simulink model "Full_load_sim_doc"  (R2020a)
settings: Solver=VariableStepAuto  StartTime=0.0  StopTime=50000  RelTol=1e-3
values from neighbouring files (symbols this model uses):
  BlySyreON = 1    [sim_starter.m]
  LiIonLilleON = 1    [sim_starter.m]
  LiIonStorON = 1    [sim_starter.m]
  LoadBlySyre = load    [sim_starter.m]
  LoadLille = load    [sim_starter.m]
  LoadLiStor = 0    [sim_starter.m]
  LoadNiMH = load    [sim_starter.m]
  LoadSaltVand = load    [sim_starter.m]
  NiMHON = 1    [sim_starter.m]
  SaltVandON = 1    [sim_starter.m]
undefined symbols (not defined in the file or in its folder): Hydride, Metal, Nickel
libraries: nesl_utility x28, fl_lib x24, powerlib x4, ee_lib x4, electricdrivelib x1
(part 1 of 2)
settings Model: PacingRate=0.100000  Creator=Philip AMH  LastModifiedBy=jenslawl
settings SolverCC: ZeroCrossAlgorithm=Adaptive  AlgebraicLoopSolver=LineSearch
settings OptimizationCC: DefaultParameterBehavior=Inlined  UseDivisionForNetSlopeComputation=on  GainParamInheritBuiltInType=on  UseFloatMulNetSlope=on  InlineInvariantSignals=on  EnhancedBackFolding=on  BooleansAsBitfields=on  PassReuseOutputArgsAs=Individual arguments  StateBitsets=on  DataBitsets=on  ZeroExternalMemoryAtStartup=off  ZeroInternalMemoryAtStartup=off  NoFixptDivByZeroProtection=on  EfficientFloat2IntCast=on  LifeSpan=1  OptimizeBlockOrder=speed  DifferentSizesBufferReuse=on  EfficientTunableParamExpr=on
settings DebuggingCC: IgnoredZcDiagnostic=none  ParameterTunabilityLossMsg=error
settings SFSimCC: MATLABDynamicMemAlloc=off
settings RTWCC: SystemTargetFile=ert.tlc  TemplateMakefile=ert_default_tmf  TargetLang=C++
settings CodeAppCC: ForceParamTrailComments=on  IgnoreCustomStorageClasses=off  OperatorAnnotations=on  SimulinkDataObjDesc=on  SFDataObjDesc=on  CustomSymbolStrGlobalVar=rt$N$M  CustomSymbolStrType=$N$M  CustomSymbolStrFcn=$N$M$F  CustomSymbolStrMacro=$N$M  InsertBlockDesc=on
settings ERTTargetCC: TargetLangStandard=C++03 (ISO)  GenerateSampleERTMain=on  IncludeMdlTerminateFcn=off  CombineSignalStateStructs=on  SupportAbsoluteTime=off  SupportComplex=off  SupportContinuousTime=on  InlinedParameterPlacement=NonHierarchical  RootIOFormat=Structure reference  ERTCustomFileTemplate=example_file_process.tlc  ERTFilePackagingFormat=CompactWithDataFile

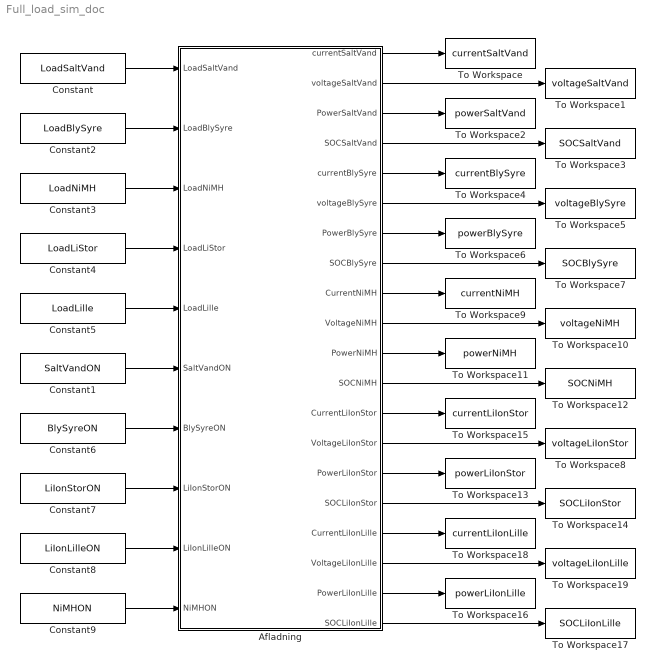
== system Full_load_sim_doc ==
  Afladning : Subsystem
  Constant : Constant  Value=LoadSaltVand
  Constant1 : Constant  Value=SaltVandON
  Constant2 : Constant  Value=LoadBlySyre
  Constant3 : Constant  Value=LoadNiMH
  Constant4 : Constant  Value=LoadLiStor
  Constant5 : Constant  Value=LoadLille
  Constant6 : Constant  Value=BlySyreON
  Constant7 : Constant  Value=LiIonStorON
  Constant8 : Constant  Value=LiIonLilleON
  Constant9 : Constant  Value=NiMHON
  To Workspace : ToWorkspace  VariableName=currentSaltVand  SampleTime=-1
  To Workspace1 : ToWorkspace  VariableName=voltageSaltVand  SampleTime=-1
  To Workspace10 : ToWorkspace  VariableName=voltageNiMH  SampleTime=-1
  To Workspace11 : ToWorkspace  VariableName=powerNiMH  SampleTime=-1
  To Workspace12 : ToWorkspace  VariableName=SOCNiMH  SampleTime=-1
  To Workspace13 : ToWorkspace  VariableName=powerLiIonStor  SampleTime=-1
  To Workspace14 : ToWorkspace  VariableName=SOCLiIonStor  SampleTime=-1
  To Workspace15 : ToWorkspace  VariableName=currentLiIonStor  SampleTime=-1
  To Workspace16 : ToWorkspace  VariableName=powerLiIonLille  SampleTime=-1
  To Workspace17 : ToWorkspace  VariableName=SOCLiIonLille  SampleTime=-1
  To Workspace18 : ToWorkspace  VariableName=currentLiIonLille  SampleTime=-1
  To Workspace19 : ToWorkspace  VariableName=voltageLiIonLille  SampleTime=-1
  To Workspace2 : ToWorkspace  VariableName=powerSaltVand  SampleTime=-1
  To Workspace3 : ToWorkspace  VariableName=SOCSaltVand  SampleTime=-1
  To Workspace4 : ToWorkspace  VariableName=currentBlySyre  SampleTime=-1
  To Workspace5 : ToWorkspace  VariableName=voltageBlySyre  SampleTime=-1
  To Workspace6 : ToWorkspace  VariableName=powerBlySyre  SampleTime=-1
  To Workspace7 : ToWorkspace  VariableName=SOCBlySyre  SampleTime=-1
  To Workspace8 : ToWorkspace  VariableName=voltageLiIonStor  SampleTime=-1
  To Workspace9 : ToWorkspace  VariableName=currentNiMH  SampleTime=-1
  wires:
  Constant/1 -> Afladning/1(LoadSaltVand)
  Constant2/1 -> Afladning/2(LoadBlySyre)
  Constant3/1 -> Afladning/3(LoadNiMH)
  Constant4/1 -> Afladning/4(LoadLiStor)
  Constant5/1 -> Afladning/5(LoadLille)
  Constant1/1 -> Afladning/6(SaltVandON)
  Constant6/1 -> Afladning/7(BlySyreON)
  Constant7/1 -> Afladning/8(LiIonStorON)
  Constant8/1 -> Afladning/9(LiIonLilleON)
  Constant9/1 -> Afladning/10(NiMHON)
  Afladning/1(currentSaltVand) -> To Workspace/1
  Afladning/3(PowerSaltVand) -> To Workspace2/1
  Afladning/2(voltageSaltVand) -> To Workspace1/1
  Afladning/4(SOCSaltVand) -> To Workspace3/1
  Afladning/8(SOCBlySyre) -> To Workspace7/1
  Afladning/6(voltageBlySyre) -> To Workspace5/1
  Afladning/5(currentBlySyre) -> To Workspace4/1
  Afladning/7(PowerBlySyre) -> To Workspace6/1
  Afladning/9(CurrentNiMH) -> To Workspace9/1
  Afladning/12(SOCNiMH) -> To Workspace12/1
  Afladning/11(PowerNiMH) -> To Workspace11/1
  Afladning/10(VoltageNiMH) -> To Workspace10/1
  Afladning/16(SOCLiIonStor) -> To Workspace14/1
  Afladning/14(VoltageLiIonStor) -> To Workspace8/1
  Afladning/13(CurrentLiIonStor) -> To Workspace15/1
  Afladning/15(PowerLiIonStor) -> To Workspace13/1
  Afladning/18(VoltageLiIonLille) -> To Workspace19/1
  Afladning/20(SOCLiIonLille) -> To Workspace17/1
  Afladning/17(CurrentLiIonLille) -> To Workspace18/1
  Afladning/19(PowerLiIonLille) -> To Workspace16/1

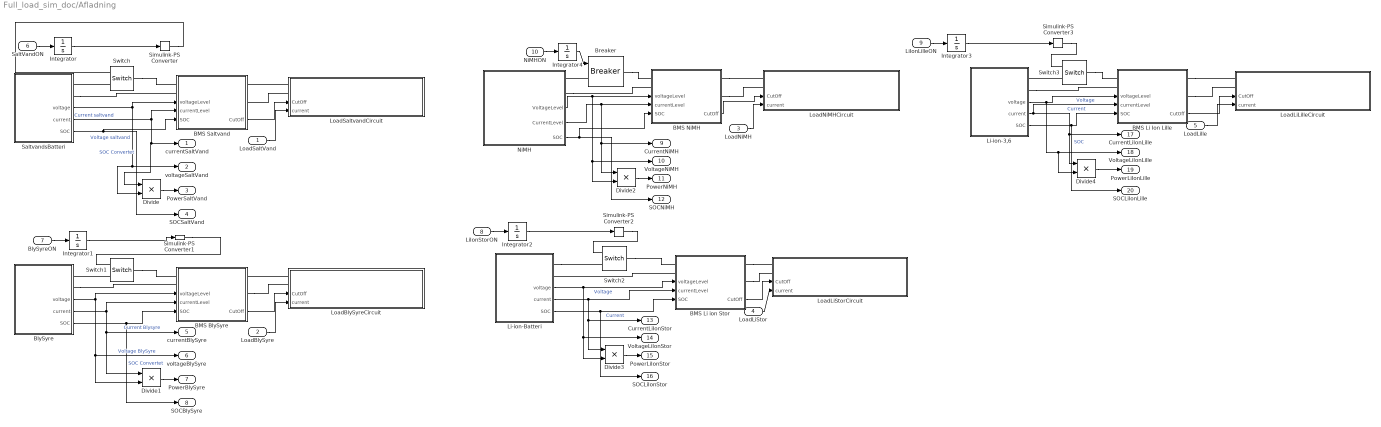
== system Full_load_sim_doc/Afladning ==
  LoadSaltVand : Inport
  LoadBlySyre : Inport  Port=2
  LoadNiMH : Inport  Port=3
  LoadLiStor : Inport  Port=4
  LoadLille : Inport  Port=5
  SaltVandON : Inport  Port=6
  BlySyreON : Inport  Port=7
  LiIonStorON : Inport  Port=8
  LiIonLilleON : Inport  Port=9
  NiMHON : Inport  Port=10
  BMS BlySyre : Subsystem
      settings: PortSchema="{\"entries\":[{\"content\":{\"sides\":[{\"content\":{\"connectorIds\":[\"LConn1\",\"LConn2\",\"In1\",\"In2\",\"In3\"]},\"type\":\"ConnectorPlacement.EquallySpacedRectSide\",\"uuid\":\"8e5b19d5-26fd-4308-a068-31d3a7110353\"},{\"content\":{\"connectorIds\":[\"RConn1\",\"RConn2\",\"Out1\"],\"side\":\"RIGHT\"},\"type\":\"ConnectorPlacement.EquallySpacedRectSide\",\"uuid\":\"43c00b24-a96d-45dd-baf7-73862471a89e\"},{\"content\":{\"connectorIds\":[],\"side\":\"TOP\"},\"type\":\"ConnectorPlacement.EquallySpacedRectSide\",\"uuid\":\"aec9a084-a9ff-4300-b99c-89bc23ebac6c\"}]},\"type\":\"ConnectorPlacement.EquallySpacedConnector\",\"uuid\":\"d767dd7e-ef5e-469c-820c-a4f5797d1fb9\"}],\"packageUris\":[\"http://schema.mathworks.com/mf0/Connector/19700101\"],\"version\":\"1.0\"}"
  BMS Li Ion Lille : Subsystem
      settings: PortSchema="{\"entries\":[{\"content\":{\"sides\":[{\"content\":{\"connectorIds\":[\"LConn1\",\"LConn2\",\"In1\",\"In2\",\"In3\"]},\"type\":\"ConnectorPlacement.EquallySpacedRectSide\",\"uuid\":\"8e5b19d5-26fd-4308-a068-31d3a7110353\"},{\"content\":{\"connectorIds\":[\"RConn1\",\"RConn2\",\"Out1\"],\"side\":\"RIGHT\"},\"type\":\"ConnectorPlacement.EquallySpacedRectSide\",\"uuid\":\"43c00b24-a96d-45dd-baf7-73862471a89e\"},{\"content\":{\"connectorIds\":[],\"side\":\"TOP\"},\"type\":\"ConnectorPlacement.EquallySpacedRectSide\",\"uuid\":\"aec9a084-a9ff-4300-b99c-89bc23ebac6c\"}]},\"type\":\"ConnectorPlacement.EquallySpacedConnector\",\"uuid\":\"d767dd7e-ef5e-469c-820c-a4f5797d1fb9\"}],\"packageUris\":[\"http://schema.mathworks.com/mf0/Connector/19700101\"],\"version\":\"1.0\"}"
  BMS Li ion Stor : Subsystem
      settings: PortSchema="{\"entries\":[{\"content\":{\"sides\":[{\"content\":{\"connectorIds\":[\"LConn1\",\"LConn2\",\"In1\",\"In2\",\"In3\"]},\"type\":\"ConnectorPlacement.EquallySpacedRectSide\",\"uuid\":\"8e5b19d5-26fd-4308-a068-31d3a7110353\"},{\"content\":{\"connectorIds\":[\"RConn1\",\"RConn2\",\"Out1\"],\"side\":\"RIGHT\"},\"type\":\"ConnectorPlacement.EquallySpacedRectSide\",\"uuid\":\"43c00b24-a96d-45dd-baf7-73862471a89e\"},{\"content\":{\"connectorIds\":[],\"side\":\"TOP\"},\"type\":\"ConnectorPlacement.EquallySpacedRectSide\",\"uuid\":\"aec9a084-a9ff-4300-b99c-89bc23ebac6c\"}]},\"type\":\"ConnectorPlacement.EquallySpacedConnector\",\"uuid\":\"d767dd7e-ef5e-469c-820c-a4f5797d1fb9\"}],\"packageUris\":[\"http://schema.mathworks.com/mf0/Connector/19700101\"],\"version\":\"1.0\"}"
  BMS NiMH : Subsystem
      settings: PortSchema="{\"entries\":[{\"content\":{\"sides\":[{\"content\":{\"connectorIds\":[\"LConn1\",\"LConn2\",\"In1\",\"In2\",\"In3\"]},\"type\":\"ConnectorPlacement.EquallySpacedRectSide\",\"uuid\":\"8e5b19d5-26fd-4308-a068-31d3a7110353\"},{\"content\":{\"connectorIds\":[\"RConn1\",\"RConn2\",\"Out1\"],\"side\":\"RIGHT\"},\"type\":\"ConnectorPlacement.EquallySpacedRectSide\",\"uuid\":\"43c00b24-a96d-45dd-baf7-73862471a89e\"},{\"content\":{\"connectorIds\":[],\"side\":\"TOP\"},\"type\":\"ConnectorPlacement.EquallySpacedRectSide\",\"uuid\":\"aec9a084-a9ff-4300-b99c-89bc23ebac6c\"}]},\"type\":\"ConnectorPlacement.EquallySpacedConnector\",\"uuid\":\"d767dd7e-ef5e-469c-820c-a4f5797d1fb9\"}],\"packageUris\":[\"http://schema.mathworks.com/mf0/Connector/19700101\"],\"version\":\"1.0\"}"
  "BMS Saltvand " : Subsystem
      settings: PortSchema="{\"entries\":[{\"content\":{\"sides\":[{\"content\":{\"connectorIds\":[\"LConn1\",\"LConn2\",\"In1\",\"In2\",\"In3\"]},\"type\":\"ConnectorPlacement.EquallySpacedRectSide\",\"uuid\":\"8e5b19d5-26fd-4308-a068-31d3a7110353\"},{\"content\":{\"connectorIds\":[\"RConn1\",\"RConn2\",\"Out1\"],\"side\":\"RIGHT\"},\"type\":\"ConnectorPlacement.EquallySpacedRectSide\",\"uuid\":\"43c00b24-a96d-45dd-baf7-73862471a89e\"},{\"content\":{\"connectorIds\":[],\"side\":\"TOP\"},\"type\":\"ConnectorPlacement.EquallySpacedRectSide\",\"uuid\":\"aec9a084-a9ff-4300-b99c-89bc23ebac6c\"}]},\"type\":\"ConnectorPlacement.EquallySpacedConnector\",\"uuid\":\"d767dd7e-ef5e-469c-820c-a4f5797d1fb9\"}],\"packageUris\":[\"http://schema.mathworks.com/mf0/Connector/19700101\"],\"version\":\"1.0\"}"
  BlySyre : Subsystem
      settings: PortSchema="{\"entries\":[{\"content\":{\"sides\":[{\"content\":{\"connectorIds\":[]},\"type\":\"ConnectorPlacement.EquallySpacedRectSide\",\"uuid\":\"b7adcffb-368c-467a-b339-3146d53f89f7\"},{\"content\":{\"connectorIds\":[\"RConn1\",\"RConn2\",\"Out1\",\"Out2\",\"Out3\"],\"side\":\"RIGHT\"},\"type\":\"ConnectorPlacement.EquallySpacedRectSide\",\"uuid\":\"78fa0dc6-8b86-442a-9e1f-c20c2cc39690\"},{\"content\":{\"connectorIds\":[],\"side\":\"TOP\"},\"type\":\"ConnectorPlacement.EquallySpacedRectSide\",\"uuid\":\"02b6bb54-52f8-4387-9821-90c0e82d6c22\"}]},\"type\":\"ConnectorPlacement.EquallySpacedConnector\",\"uuid\":\"f2eebdbf-49bd-409e-a7c0-76b4bde01873\"}],\"packageUris\":[\"http://schema.mathworks.com/mf0/Connector/19700101\"],\"version\":\"1.0\"}"
  Breaker : powerlib/Elements/Breaker  InitialState=0  SwitchingTimes="[1/60  5/60]"  External=on  BreakerResistance=0.01  SnubberResistance=1e6  SnubberCapacitance=inf  Measurements=None  MoreParameters=on  NoBreakLoop=off
  Divide{,1..4} (5 alike) : Product  Inputs=**
  Integrator{,1..4} (5 alike) : Integrator
  Li-ion-3,6 : Subsystem
      settings: PortSchema="{\"entries\":[{\"content\":{\"sides\":[{\"content\":{\"connectorIds\":[]},\"type\":\"ConnectorPlacement.EquallySpacedRectSide\",\"uuid\":\"b7adcffb-368c-467a-b339-3146d53f89f7\"},{\"content\":{\"connectorIds\":[\"RConn1\",\"RConn2\",\"Out1\",\"Out2\",\"Out3\"],\"side\":\"RIGHT\"},\"type\":\"ConnectorPlacement.EquallySpacedRectSide\",\"uuid\":\"78fa0dc6-8b86-442a-9e1f-c20c2cc39690\"},{\"content\":{\"connectorIds\":[],\"side\":\"TOP\"},\"type\":\"ConnectorPlacement.EquallySpacedRectSide\",\"uuid\":\"02b6bb54-52f8-4387-9821-90c0e82d6c22\"}]},\"type\":\"ConnectorPlacement.EquallySpacedConnector\",\"uuid\":\"f2eebdbf-49bd-409e-a7c0-76b4bde01873\"}],\"packageUris\":[\"http://schema.mathworks.com/mf0/Connector/19700101\"],\"version\":\"1.0\"}"
  Li-ion-Batteri : Subsystem
      settings: PortSchema="{\"entries\":[{\"content\":{\"sides\":[{\"content\":{\"connectorIds\":[]},\"type\":\"ConnectorPlacement.EquallySpacedRectSide\",\"uuid\":\"b7adcffb-368c-467a-b339-3146d53f89f7\"},{\"content\":{\"connectorIds\":[\"RConn1\",\"RConn2\",\"Out1\",\"Out2\",\"Out3\"],\"side\":\"RIGHT\"},\"type\":\"ConnectorPlacement.EquallySpacedRectSide\",\"uuid\":\"78fa0dc6-8b86-442a-9e1f-c20c2cc39690\"},{\"content\":{\"connectorIds\":[],\"side\":\"TOP\"},\"type\":\"ConnectorPlacement.EquallySpacedRectSide\",\"uuid\":\"02b6bb54-52f8-4387-9821-90c0e82d6c22\"}]},\"type\":\"ConnectorPlacement.EquallySpacedConnector\",\"uuid\":\"f2eebdbf-49bd-409e-a7c0-76b4bde01873\"}],\"packageUris\":[\"http://schema.mathworks.com/mf0/Connector/19700101\"],\"version\":\"1.0\"}"
  LoadBlySyreCircuit : Subsystem
      settings: PortSchema="{\"entries\":[{\"content\":{\"sides\":[{\"content\":{\"connectorIds\":[\"LConn1\",\"LConn2\",\"In1\",\"In2\"]},\"type\":\"ConnectorPlacement.EquallySpacedRectSide\",\"uuid\":\"b5cadee7-2d01-46ee-bf49-69402e8f136b\"},{\"content\":{\"connectorIds\":[],\"side\":\"RIGHT\"},\"type\":\"ConnectorPlacement.EquallySpacedRectSide\",\"uuid\":\"c93f53f5-1213-453b-bd10-619be19bd60a\"},{\"content\":{\"connectorIds\":[],\"side\":\"TOP\"},\"type\":\"ConnectorPlacement.EquallySpacedRectSide\",\"uuid\":\"b4015440-ddf2-46e7-8a1d-8162baf69575\"}]},\"type\":\"ConnectorPlacement.EquallySpacedConnector\",\"uuid\":\"d9e17d4e-0efd-4077-956a-1911f70d4ae6\"}],\"packageUris\":[\"http://schema.mathworks.com/mf0/Connector/19700101\"],\"version\":\"1.0\"}"
  LoadLiLilleCircuit : Subsystem
      settings: PortSchema="{\"entries\":[{\"content\":{\"sides\":[{\"content\":{\"connectorIds\":[\"LConn1\",\"LConn2\",\"In1\",\"In2\"]},\"type\":\"ConnectorPlacement.EquallySpacedRectSide\",\"uuid\":\"b5cadee7-2d01-46ee-bf49-69402e8f136b\"},{\"content\":{\"connectorIds\":[],\"side\":\"RIGHT\"},\"type\":\"ConnectorPlacement.EquallySpacedRectSide\",\"uuid\":\"c93f53f5-1213-453b-bd10-619be19bd60a\"},{\"content\":{\"connectorIds\":[],\"side\":\"TOP\"},\"type\":\"ConnectorPlacement.EquallySpacedRectSide\",\"uuid\":\"b4015440-ddf2-46e7-8a1d-8162baf69575\"}]},\"type\":\"ConnectorPlacement.EquallySpacedConnector\",\"uuid\":\"d9e17d4e-0efd-4077-956a-1911f70d4ae6\"}],\"packageUris\":[\"http://schema.mathworks.com/mf0/Connector/19700101\"],\"version\":\"1.0\"}"
  LoadLiStorCircuit : Subsystem
      settings: PortSchema="{\"entries\":[{\"content\":{\"sides\":[{\"content\":{\"connectorIds\":[\"LConn1\",\"LConn2\",\"In1\",\"In2\"]},\"type\":\"ConnectorPlacement.EquallySpacedRectSide\",\"uuid\":\"b5cadee7-2d01-46ee-bf49-69402e8f136b\"},{\"content\":{\"connectorIds\":[],\"side\":\"RIGHT\"},\"type\":\"ConnectorPlacement.EquallySpacedRectSide\",\"uuid\":\"c93f53f5-1213-453b-bd10-619be19bd60a\"},{\"content\":{\"connectorIds\":[],\"side\":\"TOP\"},\"type\":\"ConnectorPlacement.EquallySpacedRectSide\",\"uuid\":\"b4015440-ddf2-46e7-8a1d-8162baf69575\"}]},\"type\":\"ConnectorPlacement.EquallySpacedConnector\",\"uuid\":\"d9e17d4e-0efd-4077-956a-1911f70d4ae6\"}],\"packageUris\":[\"http://schema.mathworks.com/mf0/Connector/19700101\"],\"version\":\"1.0\"}"
  LoadNiMHCircuit : Subsystem
      settings: PortSchema="{\"entries\":[{\"content\":{\"sides\":[{\"content\":{\"connectorIds\":[\"LConn1\",\"LConn2\",\"In1\",\"In2\"]},\"type\":\"ConnectorPlacement.EquallySpacedRectSide\",\"uuid\":\"5669fcd5-486b-4108-a785-c4b9f96251dd\"},{\"content\":{\"connectorIds\":[],\"side\":\"RIGHT\"},\"type\":\"ConnectorPlacement.EquallySpacedRectSide\",\"uuid\":\"14afdab1-cccb-4425-b7d2-d38de7e69fd7\"},{\"content\":{\"connectorIds\":[],\"side\":\"TOP\"},\"type\":\"ConnectorPlacement.EquallySpacedRectSide\",\"uuid\":\"ed632fd4-9432-45fd-a52c-62cd09b0fcf3\"},{\"content\":{\"connectorIds\":[],\"side\":\"BOTTOM\"},\"type\":\"ConnectorPlacement.EquallySpacedRectSide\",\"uuid\":\"47990d72-dbcd-4900-bcb8-8e776bccb935\"}]},\"type\":\"ConnectorPlacement.EquallySpacedConnector\",\"uuid\":\"96f1cb22-e1a2-4291-b2f2-f9073f63c4bf\"}],\"packageUris\":[\"http://schema.mathworks.com/mf0/Connector/19700101\"],\"version\":\"1.0\"}"
  LoadSaltvandCircuit : Subsystem
      settings: PortSchema="{\"entries\":[{\"content\":{\"sides\":[{\"content\":{\"connectorIds\":[\"LConn1\",\"LConn2\",\"In1\",\"In2\"]},\"type\":\"ConnectorPlacement.EquallySpacedRectSide\",\"uuid\":\"b5cadee7-2d01-46ee-bf49-69402e8f136b\"},{\"content\":{\"connectorIds\":[],\"side\":\"RIGHT\"},\"type\":\"ConnectorPlacement.EquallySpacedRectSide\",\"uuid\":\"c93f53f5-1213-453b-bd10-619be19bd60a\"},{\"content\":{\"connectorIds\":[],\"side\":\"TOP\"},\"type\":\"ConnectorPlacement.EquallySpacedRectSide\",\"uuid\":\"b4015440-ddf2-46e7-8a1d-8162baf69575\"}]},\"type\":\"ConnectorPlacement.EquallySpacedConnector\",\"uuid\":\"d9e17d4e-0efd-4077-956a-1911f70d4ae6\"}],\"packageUris\":[\"http://schema.mathworks.com/mf0/Connector/19700101\"],\"version\":\"1.0\"}"
  NiMH : Subsystem
      settings: PortSchema="{\"entries\":[{\"content\":{\"sides\":[{\"content\":{\"connectorIds\":[]},\"type\":\"ConnectorPlacement.EquallySpacedRectSide\",\"uuid\":\"fc65cf16-1b08-48cf-a4b8-6124313288b7\"},{\"content\":{\"connectorIds\":[\"RConn1\",\"RConn2\",\"Out1\",\"Out2\",\"Out3\"],\"side\":\"RIGHT\"},\"type\":\"ConnectorPlacement.EquallySpacedRectSide\",\"uuid\":\"2587f880-824f-409e-889d-6e6395f8efa4\"},{\"content\":{\"connectorIds\":[],\"side\":\"TOP\"},\"type\":\"ConnectorPlacement.EquallySpacedRectSide\",\"uuid\":\"a61b6a50-66af-4684-a024-cf79c14250f1\"}]},\"type\":\"ConnectorPlacement.EquallySpacedConnector\",\"uuid\":\"60ef1120-39c0-433f-916b-5d1a9aec7516\"}],\"packageUris\":[\"http://schema.mathworks.com/mf0/Connector/19700101\"],\"version\":\"1.0\"}"
  SaltvandsBatteri : Subsystem
      settings: PortSchema="{\"entries\":[{\"content\":{\"sides\":[{\"content\":{\"connectorIds\":[]},\"type\":\"ConnectorPlacement.EquallySpacedRectSide\",\"uuid\":\"b7adcffb-368c-467a-b339-3146d53f89f7\"},{\"content\":{\"connectorIds\":[\"RConn1\",\"RConn2\",\"Out1\",\"Out2\",\"Out3\"],\"side\":\"RIGHT\"},\"type\":\"ConnectorPlacement.EquallySpacedRectSide\",\"uuid\":\"78fa0dc6-8b86-442a-9e1f-c20c2cc39690\"},{\"content\":{\"connectorIds\":[],\"side\":\"TOP\"},\"type\":\"ConnectorPlacement.EquallySpacedRectSide\",\"uuid\":\"02b6bb54-52f8-4387-9821-90c0e82d6c22\"}]},\"type\":\"ConnectorPlacement.EquallySpacedConnector\",\"uuid\":\"f2eebdbf-49bd-409e-a7c0-76b4bde01873\"}],\"packageUris\":[\"http://schema.mathworks.com/mf0/Connector/19700101\"],\"version\":\"1.0\"}"
  Simulink-PS Converter{,1..3} (4 alike) : nesl_utility/Simulink-PS Converter  PhysicalDomain=network_engine_domain  SubClassName=ps_input  LeftPortType=input  RightPortType=output  PseudoPeriodic=off  Frequencies=[]  NoiseDistribution=none  NoiseParameters=[]  Unit=V  AffineConversion=on  FilteringAndDerivatives=provide  SimscapeFilterOrder=1  InputFilterTimeConstant=0.001  UdotUserProvided=0
  Switch{,1..3} (4 alike) : fl_lib/Electrical/Electrical Elements/Switch  R_closed=0.01 Ohm  G_open=1e-8 1/Ohm  Threshold=0.5  i_specify=off  i_priority=None  i=0 A  i_nominal_specify=off  i_nominal_unit=A  i_nominal_value=1  v_specify=off  v_priority=None  v=0 V  v_nominal_specify=off  v_nominal_unit=V  v_nominal_value=1
  currentSaltVand : Outport
  voltageSaltVand : Outport  Port=2
  PowerSaltVand : Outport  Port=3
  SOCSaltVand : Outport  Port=4
  currentBlySyre : Outport  Port=5
  voltageBlySyre : Outport  Port=6
  PowerBlySyre : Outport  Port=7
  SOCBlySyre : Outport  Port=8
  CurrentNiMH : Outport  Port=9
  VoltageNiMH : Outport  Port=10
  PowerNiMH : Outport  Port=11
  SOCNiMH : Outport  Port=12
  CurrentLiIonStor : Outport  Port=13
  VoltageLiIonStor : Outport  Port=14
  PowerLiIonStor : Outport  Port=15
  SOCLiIonStor : Outport  Port=16
  CurrentLiIonLille : Outport  Port=17
  VoltageLiIonLille : Outport  Port=18
  PowerLiIonLille : Outport  Port=19
  SOCLiIonLille : Outport  Port=20
  wires:
  LiIonLilleON/1 -> Integrator3/1
  LoadBlySyre/1 -> LoadBlySyreCircuit/2(current)
  Li-ion-Batteri/3(SOC) -> SOCLiIonStor/1, BMS Li ion Stor/3(SOC)
  Integrator2/1 -> Simulink-PS Converter2/1
  "BMS Saltvand "/1(CutOff) -> LoadSaltvandCircuit/1(CutOff)
  BlySyre/3(SOC) -> SOCBlySyre/1, BMS BlySyre/3(SOC)  "SOC Convertet"
  SaltvandsBatteri/2(current) -> currentSaltVand/1, Divide/1, "BMS Saltvand "/2(currentLevel)  "Current saltvand"
  BlySyre/1(voltage) -> BMS BlySyre/1(voltageLevel), voltageBlySyre/1, Divide1/2  "Voltage BlySyre"
  BMS NiMH/1(CutOff) -> LoadNiMHCircuit/1(CutOff)
  Li-ion-3,6/1(voltage) -> BMS Li Ion Lille/1(voltageLevel), VoltageLiIonLille/1, Divide4/2  "Voltage"
  BlySyre/2(current) -> currentBlySyre/1, Divide1/1, BMS BlySyre/2(currentLevel)  "Current Blysyre"
  Li-ion-Batteri/1(voltage) -> VoltageLiIonStor/1, Divide3/2, BMS Li ion Stor/1(voltageLevel)  "Voltage"
  LiIonStorON/1 -> Integrator2/1
  SaltvandsBatteri/3(SOC) -> SOCSaltVand/1, "BMS Saltvand "/3(SOC)  "SOC Convertet"
  BMS Li ion Stor/1(CutOff) -> LoadLiStorCircuit/1(CutOff)
  LoadLiStor/1 -> LoadLiStorCircuit/2(current)
  SaltvandsBatteri/1(voltage) -> voltageSaltVand/1, Divide/2, "BMS Saltvand "/1(voltageLevel)  "Voltage saltvand"
  BMS BlySyre/1(CutOff) -> LoadBlySyreCircuit/1(CutOff)
  NiMH/3(SOC) -> SOCNiMH/1, BMS NiMH/3(SOC)
  BMS Li Ion Lille/1(CutOff) -> LoadLiLilleCircuit/1(CutOff)
  Integrator3/1 -> Simulink-PS Converter3/1
  Divide2/1 -> PowerNiMH/1
  Divide4/1 -> PowerLiIonLille/1
  Integrator1/1 -> Simulink-PS Converter1/1
  NiMH/1(VoltageLevel) -> VoltageNiMH/1, Divide2/2, BMS NiMH/1(voltageLevel)
  BlySyreON/1 -> Integrator1/1
  Li-ion-Batteri/2(current) -> CurrentLiIonStor/1, Divide3/1, BMS Li ion Stor/2(currentLevel)  "Current"
  Divide1/1 -> PowerBlySyre/1
  Li-ion-3,6/2(current) -> CurrentLiIonLille/1, Divide4/1, BMS Li Ion Lille/2(currentLevel)  "Current"
  Divide/1 -> PowerSaltVand/1
  LoadNiMH/1 -> LoadNiMHCircuit/2(current)
  LoadSaltVand/1 -> LoadSaltvandCircuit/2(current)
  NiMH/2(CurrentLevel) -> BMS NiMH/2(currentLevel), CurrentNiMH/1, Divide2/1
  Li-ion-3,6/3(SOC) -> SOCLiIonLille/1, BMS Li Ion Lille/3(SOC)  "SOC"
  Divide3/1 -> PowerLiIonStor/1
  LoadLille/1 -> LoadLiLilleCircuit/2(current)
  Integrator/1 -> Simulink-PS Converter/1
  SaltVandON/1 -> Integrator/1
  NiMHON/1 -> Integrator4/1
  Integrator4/1 -> Breaker/1
  connections:
  LoadSaltvandCircuit/LConn1 -- "BMS Saltvand "/RConn1
  Switch1/RConn2 -- BlySyre/RConn1
  BMS Li ion Stor/LConn2 -- Li-ion-Batteri/RConn2
  SaltvandsBatteri/RConn2 -- "BMS Saltvand "/LConn2
  Switch1/LConn1 -- BMS BlySyre/LConn1
  LoadSaltvandCircuit/LConn2 -- "BMS Saltvand "/RConn2
  BlySyre/RConn2 -- BMS BlySyre/LConn2
  LoadBlySyreCircuit/LConn1 -- BMS BlySyre/RConn1
  Switch/LConn1 -- "BMS Saltvand "/LConn1
  NiMH/RConn2 -- BMS NiMH/LConn2
  Switch3/LConn1 -- BMS Li Ion Lille/LConn1
  Simulink-PS Converter/RConn1 -- Switch/RConn1
  Simulink-PS Converter1/RConn1 -- Switch1/RConn1
  BMS Li ion Stor/RConn1 -- LoadLiStorCircuit/LConn1
  BMS BlySyre/RConn2 -- LoadBlySyreCircuit/LConn2
  BMS NiMH/RConn1 -- LoadNiMHCircuit/LConn1
  BMS NiMH/RConn2 -- LoadNiMHCircuit/LConn2
  Simulink-PS Converter3/RConn1 -- Switch3/RConn1
  BMS Li Ion Lille/RConn2 -- LoadLiLilleCircuit/LConn2
  Simulink-PS Converter2/RConn1 -- Switch2/RConn1
  BMS Li ion Stor/RConn2 -- LoadLiStorCircuit/LConn2
  BMS Li Ion Lille/RConn1 -- LoadLiLilleCircuit/LConn1
  Switch3/RConn2 -- Li-ion-3,6/RConn1
  Breaker/LConn1 -- NiMH/RConn1
  Breaker/RConn1 -- BMS NiMH/LConn1
  Switch/RConn2 -- SaltvandsBatteri/RConn1
  Li-ion-Batteri/RConn1 -- Switch2/RConn2
  Switch2/LConn1 -- BMS Li ion Stor/LConn1
  Li-ion-3,6/RConn2 -- BMS Li Ion Lille/LConn2

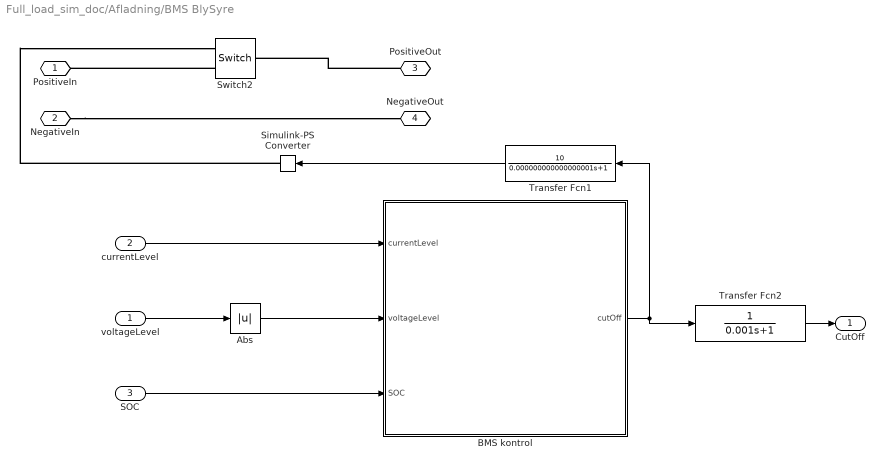
== system Full_load_sim_doc/Afladning/BMS BlySyre ==
  voltageLevel : Inport
  currentLevel : Inport  Port=2
  SOC : Inport  Port=3
  Abs : Abs
  BMS kontrol : Stateflow chart  TreatAsAtomicUnit=on
  Simulink-PS Converter : nesl_utility/Simulink-PS Converter  PhysicalDomain=network_engine_domain  SubClassName=ps_input  LeftPortType=input  RightPortType=output  PseudoPeriodic=off  Frequencies=[]  NoiseDistribution=none  NoiseParameters=[]  Unit=V  AffineConversion=off  FilteringAndDerivatives=provide  SimscapeFilterOrder=1  InputFilterTimeConstant=0.001  UdotUserProvided=0
  Switch2 : fl_lib/Electrical/Electrical Elements/Switch  R_closed=0.01 Ohm  G_open=1e-8 1/Ohm  Threshold=0.5  i_specify=off  i_priority=None  i=0 A  i_nominal_specify=off  i_nominal_unit=A  i_nominal_value=1  v_specify=off  v_priority=None  v=0 V  v_nominal_specify=off  v_nominal_unit=V  v_nominal_value=1
  Transfer Fcn1 : TransferFcn  Numerator=[10]  Denominator=[0.000000000000000001 1]
  Transfer Fcn2 : TransferFcn  Denominator=[0.001 1]
  PositiveIn : PMIOPort  Side=Left
  NegativeIn : PMIOPort  Port=2  Side=Left
  PositiveOut : PMIOPort  Port=3  Side=Right
  NegativeOut : PMIOPort  Port=4  Side=Right
  CutOff : Outport
  wires:
  SOC/1 -> BMS kontrol/3(SOC)
  BMS kontrol/1(cutOff) -> Transfer Fcn2/1, Transfer Fcn1/1
  currentLevel/1 -> BMS kontrol/1(currentLevel)
  voltageLevel/1 -> Abs/1
  Transfer Fcn1/1 -> Simulink-PS Converter/1
  Transfer Fcn2/1 -> CutOff/1
  Abs/1 -> BMS kontrol/2(voltageLevel)
  connections:
  NegativeIn/RConn1 -- NegativeOut/RConn1
  Switch2/RConn2 -- PositiveIn/RConn1
  Simulink-PS Converter/RConn1 -- Switch2/RConn1
  PositiveOut/RConn1 -- Switch2/LConn1

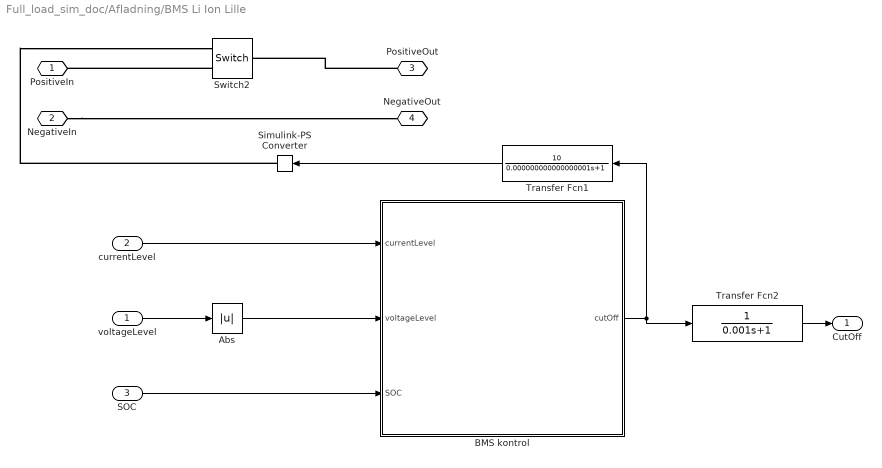
== system Full_load_sim_doc/Afladning/BMS Li Ion Lille ==
  voltageLevel : Inport
  currentLevel : Inport  Port=2
  SOC : Inport  Port=3
  Abs : Abs
  BMS kontrol : Stateflow chart  TreatAsAtomicUnit=on
  Simulink-PS Converter : nesl_utility/Simulink-PS Converter  PhysicalDomain=network_engine_domain  SubClassName=ps_input  LeftPortType=input  RightPortType=output  PseudoPeriodic=off  Frequencies=[]  NoiseDistribution=none  NoiseParameters=[]  Unit=V  AffineConversion=off  FilteringAndDerivatives=provide  SimscapeFilterOrder=1  InputFilterTimeConstant=0.001  UdotUserProvided=0
  Switch2 : fl_lib/Electrical/Electrical Elements/Switch  R_closed=0.01 Ohm  G_open=1e-8 1/Ohm  Threshold=0.5  i_specify=off  i_priority=None  i=0 A  i_nominal_specify=off  i_nominal_unit=A  i_nominal_value=1  v_specify=off  v_priority=None  v=0 V  v_nominal_specify=off  v_nominal_unit=V  v_nominal_value=1
  Transfer Fcn1 : TransferFcn  Numerator=[10]  Denominator=[0.000000000000000001 1]
  Transfer Fcn2 : TransferFcn  Denominator=[0.001 1]
  PositiveIn : PMIOPort  Side=Left
  NegativeIn : PMIOPort  Port=2  Side=Left
  PositiveOut : PMIOPort  Port=3  Side=Right
  NegativeOut : PMIOPort  Port=4  Side=Right
  CutOff : Outport
  wires:
  Transfer Fcn2/1 -> CutOff/1
  Transfer Fcn1/1 -> Simulink-PS Converter/1
  voltageLevel/1 -> Abs/1
  currentLevel/1 -> BMS kontrol/1(currentLevel)
  BMS kontrol/1(cutOff) -> Transfer Fcn1/1, Transfer Fcn2/1
  SOC/1 -> BMS kontrol/3(SOC)
  Abs/1 -> BMS kontrol/2(voltageLevel)
  connections:
  PositiveOut/RConn1 -- Switch2/LConn1
  Simulink-PS Converter/RConn1 -- Switch2/RConn1
  Switch2/RConn2 -- PositiveIn/RConn1
  NegativeIn/RConn1 -- NegativeOut/RConn1

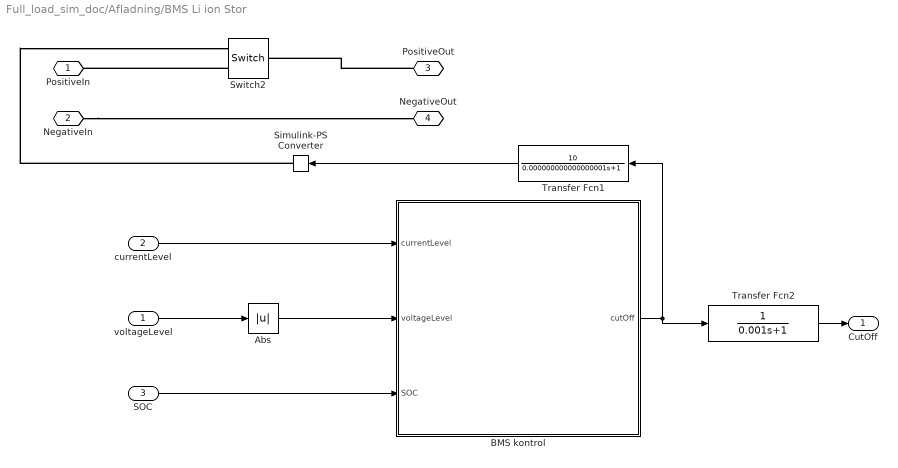
== system Full_load_sim_doc/Afladning/BMS Li ion Stor ==
  voltageLevel : Inport
  currentLevel : Inport  Port=2
  SOC : Inport  Port=3
  Abs : Abs
  BMS kontrol : Stateflow chart  TreatAsAtomicUnit=on
  Simulink-PS Converter : nesl_utility/Simulink-PS Converter  PhysicalDomain=network_engine_domain  SubClassName=ps_input  LeftPortType=input  RightPortType=output  PseudoPeriodic=off  Frequencies=[]  NoiseDistribution=none  NoiseParameters=[]  Unit=V  AffineConversion=off  FilteringAndDerivatives=provide  SimscapeFilterOrder=1  InputFilterTimeConstant=0.001  UdotUserProvided=0
  Switch2 : fl_lib/Electrical/Electrical Elements/Switch  R_closed=0.01 Ohm  G_open=1e-8 1/Ohm  Threshold=0.5  i_specify=off  i_priority=None  i=0 A  i_nominal_specify=off  i_nominal_unit=A  i_nominal_value=1  v_specify=off  v_priority=None  v=0 V  v_nominal_specify=off  v_nominal_unit=V  v_nominal_value=1
  Transfer Fcn1 : TransferFcn  Numerator=[10]  Denominator=[0.000000000000000001 1]
  Transfer Fcn2 : TransferFcn  Denominator=[0.001 1]
  PositiveIn : PMIOPort  Side=Left
  NegativeIn : PMIOPort  Port=2  Side=Left
  PositiveOut : PMIOPort  Port=3  Side=Right
  NegativeOut : PMIOPort  Port=4  Side=Right
  CutOff : Outport
  wires:
  Transfer Fcn2/1 -> CutOff/1
  Transfer Fcn1/1 -> Simulink-PS Converter/1
  voltageLevel/1 -> Abs/1
  currentLevel/1 -> BMS kontrol/1(currentLevel)
  BMS kontrol/1(cutOff) -> Transfer Fcn1/1, Transfer Fcn2/1
  SOC/1 -> BMS kontrol/3(SOC)
  Abs/1 -> BMS kontrol/2(voltageLevel)
  connections:
  PositiveOut/RConn1 -- Switch2/LConn1
  Simulink-PS Converter/RConn1 -- Switch2/RConn1
  Switch2/RConn2 -- PositiveIn/RConn1
  NegativeIn/RConn1 -- NegativeOut/RConn1

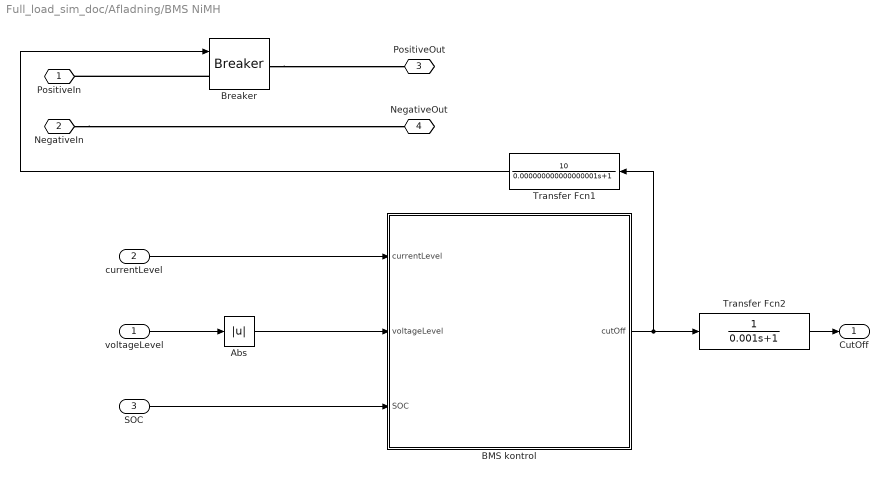
== system Full_load_sim_doc/Afladning/BMS NiMH ==
  voltageLevel : Inport
  currentLevel : Inport  Port=2
  SOC : Inport  Port=3
  Abs : Abs
  BMS kontrol : Stateflow chart  TreatAsAtomicUnit=on
  Breaker : powerlib/Elements/Breaker  InitialState=1  SwitchingTimes="[1/60  5/60]"  External=on  BreakerResistance=0.01  SnubberResistance=1e6  SnubberCapacitance=inf  Measurements=None  MoreParameters=on  NoBreakLoop=off
  Transfer Fcn1 : TransferFcn  Numerator=[10]  Denominator=[0.000000000000000001 1]
  Transfer Fcn2 : TransferFcn  Denominator=[0.001 1]
  PositiveIn : PMIOPort  Side=Left
  NegativeIn : PMIOPort  Port=2  Side=Left
  PositiveOut : PMIOPort  Port=3  Side=Right
  NegativeOut : PMIOPort  Port=4  Side=Right
  CutOff : Outport
  wires:
  Transfer Fcn2/1 -> CutOff/1
  Transfer Fcn1/1 -> Breaker/1
  voltageLevel/1 -> Abs/1
  currentLevel/1 -> BMS kontrol/1(currentLevel)
  BMS kontrol/1(cutOff) -> Transfer Fcn1/1, Transfer Fcn2/1
  SOC/1 -> BMS kontrol/3(SOC)
  Abs/1 -> BMS kontrol/2(voltageLevel)
  connections:
  NegativeIn/RConn1 -- NegativeOut/RConn1
  Breaker/LConn1 -- PositiveIn/RConn1
  Breaker/RConn1 -- PositiveOut/RConn1

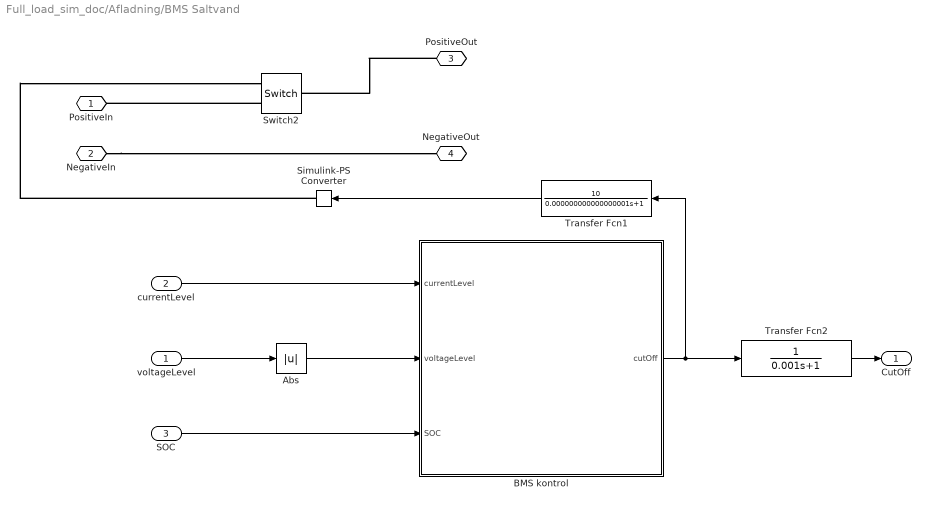
== system Full_load_sim_doc/Afladning/BMS Saltvand  ==
  voltageLevel : Inport
  currentLevel : Inport  Port=2
  SOC : Inport  Port=3
  Abs : Abs
  BMS kontrol : Stateflow chart  TreatAsAtomicUnit=on
  Simulink-PS Converter : nesl_utility/Simulink-PS Converter  PhysicalDomain=network_engine_domain  SubClassName=ps_input  LeftPortType=input  RightPortType=output  PseudoPeriodic=off  Frequencies=[]  NoiseDistribution=none  NoiseParameters=[]  Unit=V  AffineConversion=off  FilteringAndDerivatives=provide  SimscapeFilterOrder=1  InputFilterTimeConstant=0.001  UdotUserProvided=0
  Switch2 : fl_lib/Electrical/Electrical Elements/Switch  R_closed=0.01 Ohm  G_open=1e-8 1/Ohm  Threshold=0.5  i_specify=off  i_priority=None  i=0 A  i_nominal_specify=off  i_nominal_unit=A  i_nominal_value=1  v_specify=off  v_priority=None  v=0 V  v_nominal_specify=off  v_nominal_unit=V  v_nominal_value=1
  Transfer Fcn1 : TransferFcn  Numerator=[10]  Denominator=[0.000000000000000001 1]
  Transfer Fcn2 : TransferFcn  Denominator=[0.001 1]
  PositiveIn : PMIOPort  Side=Left
  NegativeIn : PMIOPort  Port=2  Side=Left
  PositiveOut : PMIOPort  Port=3  Side=Right
  NegativeOut : PMIOPort  Port=4  Side=Right
  CutOff : Outport
  wires:
  SOC/1 -> BMS kontrol/3(SOC)
  BMS kontrol/1(cutOff) -> Transfer Fcn1/1, Transfer Fcn2/1
  currentLevel/1 -> BMS kontrol/1(currentLevel)
  voltageLevel/1 -> Abs/1
  Transfer Fcn1/1 -> Simulink-PS Converter/1
  Transfer Fcn2/1 -> CutOff/1
  Abs/1 -> BMS kontrol/2(voltageLevel)
  connections:
  NegativeIn/RConn1 -- NegativeOut/RConn1
  Switch2/RConn2 -- PositiveIn/RConn1
  Simulink-PS Converter/RConn1 -- Switch2/RConn1
  PositiveOut/RConn1 -- Switch2/LConn1

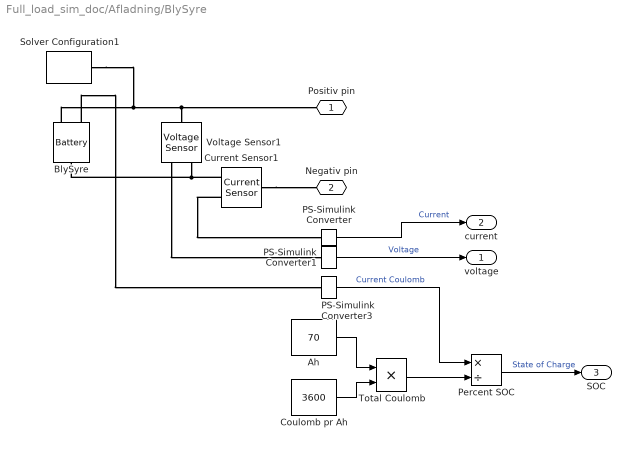
== system Full_load_sim_doc/Afladning/BlySyre ==
  Ah : Constant  Value=70
  BlySyre : ee_lib/Sources/Battery  Vnom=12 V  R1=0.001 Ohm  prm_AH=2  AH=70 hr*A  V1=10.8 V  AH1=35 hr*A  prm_R2=2  R2=2.47 kOhm  prm_dyn=2  Rp1=0.0007 Ohm  tau1=5000 s  Rp2=0.007 Ohm  tau2=50 s  Rp3=0.005 Ohm  tau3=30 s  Rp4=0.005 Ohm  tau4=30 s  Rp5=0.005 Ohm  tau5=30 s  prm_fade=2  N_fade=200  AH_fade=56 hr*A  R1_fade=2.02 Ohm  V1_fade=10.35 V  i_specify=off  i_priority=None  i=0 A  i_nominal_specify=off  i_nominal_unit=A  i_nominal_value=1  v_specify=off  v_priority=None  v=0 V  v_nominal_specify=off  v_nominal_unit=V  v_nominal_value=1  charge_specify=on  charge_priority=High  charge=70 hr*A  charge_nominal_specify=off  charge_nominal_unit=hr*A  charge_nominal_value=1  num_cycles_specify=off  num_cycles_priority=High  num_cycles=0  num_cycles_nominal_specify=off  num_cycles_nominal_unit=1  num_cycles_nominal_value=1  thermal_mass=30000 J/K  Tmeas=298.15 K  Vnom_T2=12 V  R1_T2=2.2 Ohm  V1_T2=11.4 V  R2_T2=2200 Ohm  Rp1_T2=0.005 Ohm  tau1_T2=30 s  Rp2_T2=0.005 Ohm  tau2_T2=30 s  Rp3_T2=0.005 Ohm  tau3_T2=30 s  Rp4_T2=0.005 Ohm  tau4_T2=30 s  Rp5_T2=0.005 Ohm  tau5_T2=30 s  Tmeas2=273.15 K  temperature_specify=off  temperature_priority=High  temperature=298.15 K  temperature_nominal_specify=off  temperature_nominal_unit=K  temperature_nominal_value=1
      settings: InternalSimscapePortConfiguration="{\"Bottom\":[],\"Left\":[{\"id\":\"p\",\"label\":\"+\",\"type\":\"foundation.electrical.electrical\"},{\"id\":\"q\",\"label\":\"q\",\"type\":\"output\"}],\"Right\":[{\"id\":\"n\",\"label\":\"-\",\"type\":\"foundation.electrical.electrical\"}],\"Top\":[]}"
  Coulomb pr Ah : Constant  Value=3600
  Current Sensor1 : fl_lib/Electrical/Electrical Sensors/Current Sensor
  PS-Simulink Converter : nesl_utility/PS-Simulink Converter  PhysicalDomain=network_engine_domain  SubClassName=ps_output  LeftPortType=input  RightPortType=output  PseudoPeriodic=off  Frequencies=[]  Unit=inherit  AffineConversion=off
  PS-Simulink Converter1 : nesl_utility/PS-Simulink Converter  PhysicalDomain=network_engine_domain  SubClassName=ps_output  LeftPortType=input  RightPortType=output  PseudoPeriodic=off  Frequencies=[]  Unit=inherit  AffineConversion=off
  PS-Simulink Converter3 : nesl_utility/PS-Simulink Converter  PhysicalDomain=network_engine_domain  SubClassName=ps_output  LeftPortType=input  RightPortType=output  PseudoPeriodic=off  Frequencies=[]  Unit=inherit  AffineConversion=off
  Percent SOC : Product  Inputs=*/
  Solver Configuration1 : nesl_utility/Solver Configuration  PhysicalDomain=network_engine_domain  SubClassName=solver  LeftPortType=input  RightPortType=generic  Tones=[]  Harmonics=[]  SimulateNoise=off  Profile=off  UseLocalSampling=off  EnableSwitchedLinearOptims=on  FrequencyDomain=off  UseCCode=off  RelTol=0.001  AbsTol=1e-06  MinStep=1e-09  ToWorkspace=off  RevertToSquareIcSolve=off  NumHomotopyIterations=100  PhasorMode=off  PhasorModeNumHarmonics=1  DoDC=off  ResidualTolerance=1e-09  UseLocalSolver=off  LocalSolverChoice=NE_BACKWARD_EULER_ADVANCER  LocalSolverSampleTime=0.001  DoFixedCost=off  MaxNonlinIter=3  MaxModeIter=2  LinearAlgebra=auto  EquationFormulation=NE_TIME_EF  DelaysMemoryBudget=1024  AutomaticFiltering=on  FilteringTimeConstant=0.001  PartitionStorageMethod=AS_NEEDED  PartitionMemoryBudget=1024  PartitionMethod=ROBUST
  Total Coulomb : Product  Inputs=**
  Voltage Sensor1 : fl_lib/Electrical/Electrical Sensors/Voltage Sensor
  Positiv pin : PMIOPort  Side=Right
  Negativ pin : PMIOPort  Port=2  Side=Right
  voltage : Outport
  current : Outport  Port=2
  SOC : Outport  Port=3
  wires:
  PS-Simulink Converter/1 -> current/1  "Current"
  PS-Simulink Converter1/1 -> voltage/1  "Voltage"
  Coulomb pr Ah/1 -> Total Coulomb/2
  Percent SOC/1 -> SOC/1  "State of Charge"
  PS-Simulink Converter3/1 -> Percent SOC/1  "Current Coulomb"
  Ah/1 -> Total Coulomb/1
  Total Coulomb/1 -> Percent SOC/2
  connections:
  Voltage Sensor1/RConn2 -- BlySyre/RConn1 -- Current Sensor1/RConn2
  BlySyre/LConn1 -- Positiv pin/RConn1 -- Voltage Sensor1/LConn1 -- Solver Configuration1/RConn1
  Current Sensor1/LConn1 -- Negativ pin/RConn1
  Current Sensor1/RConn1 -- PS-Simulink Converter/LConn1
  Voltage Sensor1/RConn1 -- PS-Simulink Converter1/LConn1
  BlySyre/LConn2 -- PS-Simulink Converter3/LConn1

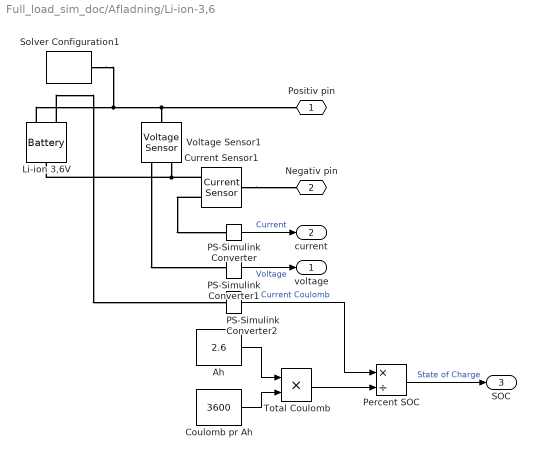
== system Full_load_sim_doc/Afladning/Li-ion-3,6 ==
  Ah : Constant  Value=2.6
  Coulomb pr Ah : Constant  Value=3600
  Current Sensor1 : fl_lib/Electrical/Electrical Sensors/Current Sensor
  Li-ion 3,6V : ee_lib/Sources/Battery  Vnom=3.7 V  R1=0.07 Ohm  prm_AH=2  AH=2.6 hr*A  V1=3.2 V  AH1=0.52 hr*A  prm_R2=1  R2=5000 Ohm  prm_dyn=3  Rp1=0.0063 Ohm  tau1=111 s  Rp2=0.0043 Ohm  tau2=111 s  Rp3=0.005 Ohm  tau3=30 s  Rp4=0.005 Ohm  tau4=30 s  Rp5=0.005 Ohm  tau5=30 s  prm_fade=2  N_fade=300  AH_fade=2.08 hr*A  R1_fade=1.084 Ohm  V1_fade=0.208 V  i_specify=off  i_priority=None  i=0 A  i_nominal_specify=off  i_nominal_unit=A  i_nominal_value=1  v_specify=off  v_priority=None  v=0 V  v_nominal_specify=off  v_nominal_unit=V  v_nominal_value=1  charge_specify=on  charge_priority=High  charge=2.6 hr*A  charge_nominal_specify=off  charge_nominal_unit=hr*A  charge_nominal_value=1  num_cycles_specify=off  num_cycles_priority=High  num_cycles=0  num_cycles_nominal_specify=off  num_cycles_nominal_unit=1  num_cycles_nominal_value=1  thermal_mass=30000 J/K  Tmeas=298.15 K  Vnom_T2=12 V  R1_T2=2.2 Ohm  V1_T2=11.4 V  R2_T2=2200 Ohm  Rp1_T2=0.005 Ohm  tau1_T2=30 s  Rp2_T2=0.005 Ohm  tau2_T2=30 s  Rp3_T2=0.005 Ohm  tau3_T2=30 s  Rp4_T2=0.005 Ohm  tau4_T2=30 s  Rp5_T2=0.005 Ohm  tau5_T2=30 s  Tmeas2=273.15 K  temperature_specify=off  temperature_priority=High  temperature=298.15 K  temperature_nominal_specify=off  temperature_nominal_unit=K  temperature_nominal_value=1
      settings: InternalSimscapePortConfiguration="{\"Bottom\":[],\"Left\":[{\"id\":\"p\",\"label\":\"+\",\"type\":\"foundation.electrical.electrical\"},{\"id\":\"q\",\"label\":\"q\",\"type\":\"output\"}],\"Right\":[{\"id\":\"n\",\"label\":\"-\",\"type\":\"foundation.electrical.electrical\"}],\"Top\":[]}"
  PS-Simulink Converter : nesl_utility/PS-Simulink Converter  PhysicalDomain=network_engine_domain  SubClassName=ps_output  LeftPortType=input  RightPortType=output  PseudoPeriodic=off  Frequencies=[]  Unit=inherit  AffineConversion=off
  PS-Simulink Converter1 : nesl_utility/PS-Simulink Converter  PhysicalDomain=network_engine_domain  SubClassName=ps_output  LeftPortType=input  RightPortType=output  PseudoPeriodic=off  Frequencies=[]  Unit=inherit  AffineConversion=off
  PS-Simulink Converter2 : nesl_utility/PS-Simulink Converter  PhysicalDomain=network_engine_domain  SubClassName=ps_output  LeftPortType=input  RightPortType=output  PseudoPeriodic=off  Frequencies=[]  Unit=inherit  AffineConversion=off
  Percent SOC : Product  Inputs=*/
  Solver Configuration1 : nesl_utility/Solver Configuration  PhysicalDomain=network_engine_domain  SubClassName=solver  LeftPortType=input  RightPortType=generic  Tones=[]  Harmonics=[]  SimulateNoise=off  Profile=off  UseLocalSampling=off  EnableSwitchedLinearOptims=on  FrequencyDomain=off  UseCCode=off  RelTol=0.001  AbsTol=1e-06  MinStep=1e-09  ToWorkspace=off  RevertToSquareIcSolve=off  NumHomotopyIterations=100  PhasorMode=off  PhasorModeNumHarmonics=1  DoDC=off  ResidualTolerance=1e-09  UseLocalSolver=off  LocalSolverChoice=NE_BACKWARD_EULER_ADVANCER  LocalSolverSampleTime=0.001  DoFixedCost=off  MaxNonlinIter=3  MaxModeIter=2  LinearAlgebra=auto  EquationFormulation=NE_TIME_EF  DelaysMemoryBudget=1024  AutomaticFiltering=on  FilteringTimeConstant=0.001  PartitionStorageMethod=AS_NEEDED  PartitionMemoryBudget=1024  PartitionMethod=ROBUST
  Total Coulomb : Product  Inputs=**
  Voltage Sensor1 : fl_lib/Electrical/Electrical Sensors/Voltage Sensor
  Positiv pin : PMIOPort  Side=Right
  Negativ pin : PMIOPort  Port=2  Side=Right
  voltage : Outport
  current : Outport  Port=2
  SOC : Outport  Port=3
  wires:
  PS-Simulink Converter/1 -> current/1  "Current"
  PS-Simulink Converter1/1 -> voltage/1  "Voltage"
  Total Coulomb/1 -> Percent SOC/2
  Percent SOC/1 -> SOC/1  "State of Charge"
  Ah/1 -> Total Coulomb/1
  PS-Simulink Converter2/1 -> Percent SOC/1  "Current Coulomb"
  Coulomb pr Ah/1 -> Total Coulomb/2
  connections:
  Voltage Sensor1/RConn2 -- Li-ion 3,6V/RConn1 -- Current Sensor1/RConn2
  Li-ion 3,6V/LConn1 -- Positiv pin/RConn1 -- Voltage Sensor1/LConn1 -- Solver Configuration1/RConn1
  Current Sensor1/LConn1 -- Negativ pin/RConn1
  Current Sensor1/RConn1 -- PS-Simulink Converter/LConn1
  Voltage Sensor1/RConn1 -- PS-Simulink Converter1/LConn1
  Li-ion 3,6V/LConn2 -- PS-Simulink Converter2/LConn1

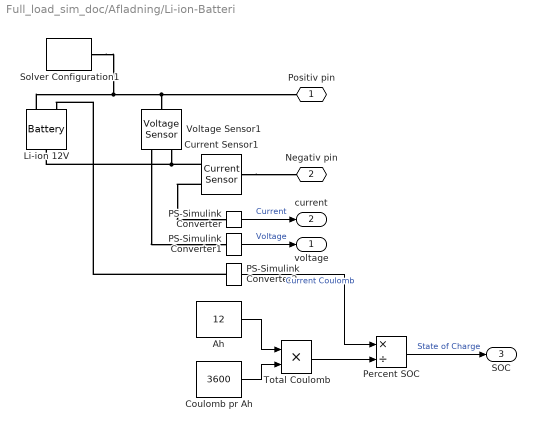
== system Full_load_sim_doc/Afladning/Li-ion-Batteri ==
  Ah : Constant  Value=12
  Coulomb pr Ah : Constant  Value=3600
  Current Sensor1 : fl_lib/Electrical/Electrical Sensors/Current Sensor
  Li-ion 12V : ee_lib/Sources/Battery  Vnom=12.8 V  R1=0.05 Ohm  prm_AH=2  AH=12 hr*A  V1=10.8 V  AH1=2 hr*A  prm_R2=1  R2=5000 Ohm  prm_dyn=3  Rp1=0.0063 Ohm  tau1=111 s  Rp2=0.0043 Ohm  tau2=111 s  Rp3=0.005 Ohm  tau3=30 s  Rp4=0.005 Ohm  tau4=30 s  Rp5=0.005 Ohm  tau5=30 s  prm_fade=2  N_fade=3000  AH_fade=10.2 hr*A  R1_fade=0.0575 Ohm  V1_fade=9.18 V  i_specify=off  i_priority=None  i=0 A  i_nominal_specify=off  i_nominal_unit=A  i_nominal_value=1  v_specify=off  v_priority=None  v=0 V  v_nominal_specify=off  v_nominal_unit=V  v_nominal_value=1  charge_specify=on  charge_priority=High  charge=12 hr*A  charge_nominal_specify=off  charge_nominal_unit=hr*A  charge_nominal_value=1  num_cycles_specify=off  num_cycles_priority=High  num_cycles=0  num_cycles_nominal_specify=off  num_cycles_nominal_unit=1  num_cycles_nominal_value=1  thermal_mass=30000 J/K  Tmeas=298.15 K  Vnom_T2=12 V  R1_T2=2.2 Ohm  V1_T2=11.4 V  R2_T2=2200 Ohm  Rp1_T2=0.005 Ohm  tau1_T2=30 s  Rp2_T2=0.005 Ohm  tau2_T2=30 s  Rp3_T2=0.005 Ohm  tau3_T2=30 s  Rp4_T2=0.005 Ohm  tau4_T2=30 s  Rp5_T2=0.005 Ohm  tau5_T2=30 s  Tmeas2=273.15 K  temperature_specify=off  temperature_priority=High  temperature=298.15 K  temperature_nominal_specify=off  temperature_nominal_unit=K  temperature_nominal_value=1
      settings: InternalSimscapePortConfiguration="{\"Bottom\":[],\"Left\":[{\"id\":\"p\",\"label\":\"+\",\"type\":\"foundation.electrical.electrical\"},{\"id\":\"q\",\"label\":\"q\",\"type\":\"output\"}],\"Right\":[{\"id\":\"n\",\"label\":\"-\",\"type\":\"foundation.electrical.electrical\"}],\"Top\":[]}"
  PS-Simulink Converter : nesl_utility/PS-Simulink Converter  PhysicalDomain=network_engine_domain  SubClassName=ps_output  LeftPortType=input  RightPortType=output  PseudoPeriodic=off  Frequencies=[]  Unit=inherit  AffineConversion=off
  PS-Simulink Converter1 : nesl_utility/PS-Simulink Converter  PhysicalDomain=network_engine_domain  SubClassName=ps_output  LeftPortType=input  RightPortType=output  PseudoPeriodic=off  Frequencies=[]  Unit=inherit  AffineConversion=off
  PS-Simulink Converter2 : nesl_utility/PS-Simulink Converter  PhysicalDomain=network_engine_domain  SubClassName=ps_output  LeftPortType=input  RightPortType=output  PseudoPeriodic=off  Frequencies=[]  Unit=inherit  AffineConversion=off
  Percent SOC : Product  Inputs=*/
  Solver Configuration1 : nesl_utility/Solver Configuration  PhysicalDomain=network_engine_domain  SubClassName=solver  LeftPortType=input  RightPortType=generic  Tones=[]  Harmonics=[]  SimulateNoise=off  Profile=off  UseLocalSampling=off  EnableSwitchedLinearOptims=on  FrequencyDomain=off  UseCCode=off  RelTol=0.001  AbsTol=1e-06  MinStep=1e-09  ToWorkspace=off  RevertToSquareIcSolve=off  NumHomotopyIterations=100  PhasorMode=off  PhasorModeNumHarmonics=1  DoDC=off  ResidualTolerance=1e-09  UseLocalSolver=off  LocalSolverChoice=NE_BACKWARD_EULER_ADVANCER  LocalSolverSampleTime=0.001  DoFixedCost=off  MaxNonlinIter=3  MaxModeIter=2  LinearAlgebra=auto  EquationFormulation=NE_TIME_EF  DelaysMemoryBudget=1024  AutomaticFiltering=on  FilteringTimeConstant=0.001  PartitionStorageMethod=AS_NEEDED  PartitionMemoryBudget=1024  PartitionMethod=ROBUST
  Total Coulomb : Product  Inputs=**
  Voltage Sensor1 : fl_lib/Electrical/Electrical Sensors/Voltage Sensor
  Positiv pin : PMIOPort  Side=Right
  Negativ pin : PMIOPort  Port=2  Side=Right
  voltage : Outport
  current : Outport  Port=2
  SOC : Outport  Port=3
  wires:
  PS-Simulink Converter/1 -> current/1  "Current"
  PS-Simulink Converter1/1 -> voltage/1  "Voltage"
  Percent SOC/1 -> SOC/1  "State of Charge"
  Coulomb pr Ah/1 -> Total Coulomb/2
  PS-Simulink Converter2/1 -> Percent SOC/1  "Current Coulomb"
  Ah/1 -> Total Coulomb/1
  Total Coulomb/1 -> Percent SOC/2
  connections:
  Voltage Sensor1/RConn2 -- Li-ion 12V/RConn1 -- Current Sensor1/RConn2
  Li-ion 12V/LConn1 -- Positiv pin/RConn1 -- Voltage Sensor1/LConn1 -- Solver Configuration1/RConn1
  Current Sensor1/LConn1 -- Negativ pin/RConn1
  Current Sensor1/RConn1 -- PS-Simulink Converter/LConn1
  Voltage Sensor1/RConn1 -- PS-Simulink Converter1/LConn1
  PS-Simulink Converter2/LConn1 -- Li-ion 12V/LConn2

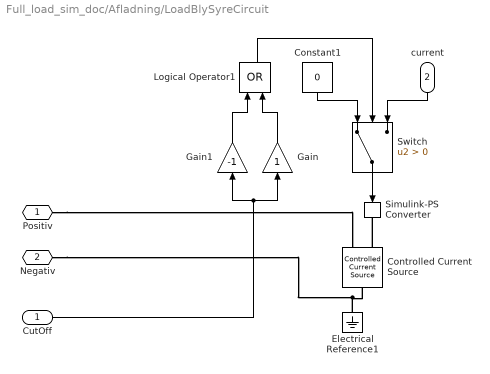
== system Full_load_sim_doc/Afladning/LoadBlySyreCircuit ==
  CutOff : Inport
  current : Inport  Port=2
  Constant1 : Constant  Value=0
  Controlled Current Source : fl_lib/Electrical/Electrical Sources/Controlled Current Source
  Electrical Reference1 : fl_lib/Electrical/Electrical Elements/Electrical Reference
  Gain : Gain
  Gain1 : Gain  Gain=-1
  Logical Operator1 : Logic  Operator=OR  AllPortsSameDT=off  OutDataTypeStr=boolean
  Simulink-PS Converter : nesl_utility/Simulink-PS Converter  PhysicalDomain=network_engine_domain  SubClassName=ps_input  LeftPortType=input  RightPortType=output  PseudoPeriodic=off  Frequencies=[]  NoiseDistribution=none  NoiseParameters=[]  Unit=1  AffineConversion=off  FilteringAndDerivatives=provide  SimscapeFilterOrder=1  InputFilterTimeConstant=0.001  UdotUserProvided=0
  Switch : Switch  Criteria=u2 > Threshold
  Positiv : PMIOPort  Side=Left
  Negativ : PMIOPort  Port=2  Side=Left
  wires:
  Gain/1 -> Logical Operator1/2
  Constant1/1 -> Switch/1
  Gain1/1 -> Logical Operator1/1
  CutOff/1 -> Gain1/1, Gain/1
  current/1 -> Switch/3
  Logical Operator1/1 -> Switch/2
  Switch/1 -> Simulink-PS Converter/1
  connections:
  Negativ/RConn1 -- Electrical Reference1/LConn1 -- Controlled Current Source/LConn1
  Controlled Current Source/RConn1 -- Simulink-PS Converter/RConn1
  Positiv/RConn1 -- Controlled Current Source/RConn2

== system Full_load_sim_doc/Afladning/LoadLiLilleCircuit ==
  CutOff : Inport
  current : Inport  Port=2
  Constant1 : Constant  Value=0
  Controlled Current Source : fl_lib/Electrical/Electrical Sources/Controlled Current Source
  Electrical Reference1 : fl_lib/Electrical/Electrical Elements/Electrical Reference
  Gain : Gain
  Gain1 : Gain  Gain=-1
  Logical Operator1 : Logic  Operator=OR  AllPortsSameDT=off  OutDataTypeStr=boolean
  Simulink-PS Converter : nesl_utility/Simulink-PS Converter  PhysicalDomain=network_engine_domain  SubClassName=ps_input  LeftPortType=input  RightPortType=output  PseudoPeriodic=off  Frequencies=[]  NoiseDistribution=none  NoiseParameters=[]  Unit=1  AffineConversion=off  FilteringAndDerivatives=provide  SimscapeFilterOrder=1  InputFilterTimeConstant=0.001  UdotUserProvided=0
  Switch : Switch  Criteria=u2 > Threshold
  Positiv : PMIOPort  Side=Left
  Negativ : PMIOPort  Port=2  Side=Left
  wires:
  Switch/1 -> Simulink-PS Converter/1
  Logical Operator1/1 -> Switch/2
  current/1 -> Switch/3
  CutOff/1 -> Gain/1, Gain1/1
  Gain1/1 -> Logical Operator1/1
  Constant1/1 -> Switch/1
  Gain/1 -> Logical Operator1/2
  connections:
  Positiv/RConn1 -- Controlled Current Source/RConn2
  Controlled Current Source/RConn1 -- Simulink-PS Converter/RConn1
  Controlled Current Source/LConn1 -- Electrical Reference1/LConn1 -- Negativ/RConn1

== system Full_load_sim_doc/Afladning/LoadLiStorCircuit ==
  CutOff : Inport
  current : Inport  Port=2
  Constant1 : Constant  Value=0
  Controlled Current Source : fl_lib/Electrical/Electrical Sources/Controlled Current Source
  Electrical Reference1 : fl_lib/Electrical/Electrical Elements/Electrical Reference
  Gain : Gain
  Gain1 : Gain  Gain=-1
  Logical Operator1 : Logic  Operator=OR  AllPortsSameDT=off  OutDataTypeStr=boolean
  Simulink-PS Converter : nesl_utility/Simulink-PS Converter  PhysicalDomain=network_engine_domain  SubClassName=ps_input  LeftPortType=input  RightPortType=output  PseudoPeriodic=off  Frequencies=[]  NoiseDistribution=none  NoiseParameters=[]  Unit=1  AffineConversion=off  FilteringAndDerivatives=provide  SimscapeFilterOrder=1  InputFilterTimeConstant=0.001  UdotUserProvided=0
  Switch : Switch  Criteria=u2 > Threshold
  Positiv : PMIOPort  Side=Left
  Negativ : PMIOPort  Port=2  Side=Left
  wires:
  Switch/1 -> Simulink-PS Converter/1
  Logical Operator1/1 -> Switch/2
  current/1 -> Switch/3
  CutOff/1 -> Gain/1, Gain1/1
  Gain1/1 -> Logical Operator1/1
  Constant1/1 -> Switch/1
  Gain/1 -> Logical Operator1/2
  connections:
  Positiv/RConn1 -- Controlled Current Source/RConn2
  Controlled Current Source/RConn1 -- Simulink-PS Converter/RConn1
  Controlled Current Source/LConn1 -- Electrical Reference1/LConn1 -- Negativ/RConn1

== system Full_load_sim_doc/Afladning/LoadNiMHCircuit ==
  CutOff : Inport
  current : Inport  Port=2
  Constant2 : Constant  Value=0
  Controlled Current Source : powerlib/Electrical Sources/Controlled Current Source  Initialize=on  Source_Type=AC  Amplitude=0  Phase=0  Frequency=0  Measurements=None
  Gain : Gain
  Gain1 : Gain  Gain=-1
  Logical Operator1 : Logic  Operator=OR  AllPortsSameDT=off  OutDataTypeStr=boolean
  Switch : Switch  Criteria=u2 > Threshold
  Positiv : PMIOPort  Side=Left
  Negativ : PMIOPort  Port=2  Side=Left
  wires:
  Switch/1 -> Controlled Current Source/1
  Gain1/1 -> Logical Operator1/1
  Gain/1 -> Logical Operator1/2
  Logical Operator1/1 -> Switch/2
  Constant2/1 -> Switch/1
  CutOff/1 -> Gain1/1, Gain/1
  current/1 -> Switch/3
  connections:
  Positiv/RConn1 -- Controlled Current Source/LConn1
  Negativ/RConn1 -- Controlled Current Source/RConn1
